simulink model "Simulink_linear_model"  (R2023b)
settings: Solver=ode45  StartTime=0.0  StopTime=10  MaxStep=0.01  RelTol=1e-3
values from neighbouring files (symbols this model uses):
  A = [0, 1,                    0, 0 ... (first row only)    [LQR_for_simscape_multibody_simulation.m]    (also in LQR_for_simulink.m)
  B = [0; (m*lc^2+J)/Delta; 0; -m*lc/Delta]    [LQR_for_simscape_multibody_simulation.m]    (also in LQR_for_simulink.m)
  K_lqr = lqr(A, B, Q, R)    [LQR_for_simscape_multibody_simulation.m]    (also in LQR_for_simulink.m)
settings Model: Creator=amira  LastModifiedBy=amira
settings DataIOCC: ReturnWorkspaceOutputs=off

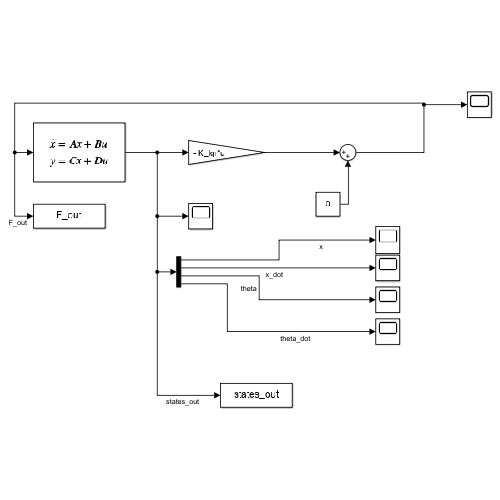
[thumbnail: Simulink's stored preview of the top-level diagram]
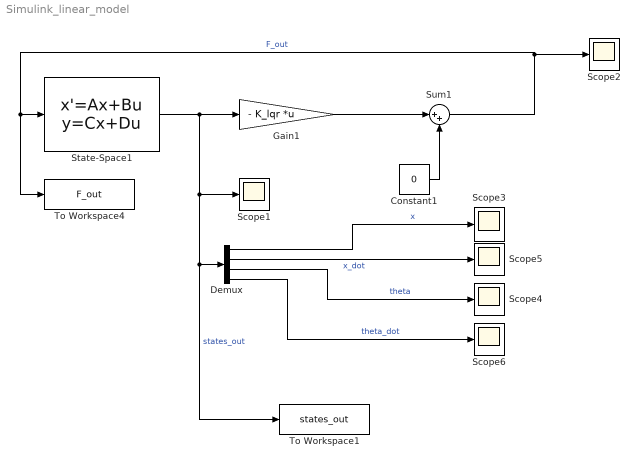
== system Simulink_linear_model ==
  Constant1 : Constant  Value=0
  Demux : Demux
  Gain1 : Gain  Gain=- K_lqr  Multiplication=Matrix(K*u)
  Scope{1..6} (6 alike) : Scope
  State-Space1 : StateSpace  A=A  B=B  C=eye(4)  D=zeros(4,1)  InitialCondition=[0; 0; 0.1; 0]  ParameterTunability=Unconstrained
  Sum1 : Sum  Inputs=|++
  To Workspace1 : ToWorkspace  VariableName=states_out  SampleTime=-1
  To Workspace4 : ToWorkspace  VariableName=F_out  SampleTime=-1
  wires:
  Constant1/1 -> Sum1/2
  Gain1/1 -> Sum1/1
  State-Space1/1 -> To Workspace1/1, Demux/1, Scope1/1, Gain1/1  "states_out"
  Demux/1 -> Scope3/1  "x"
  Demux/2 -> Scope5/1  "x_dot"
  Demux/3 -> Scope4/1  "theta"
  Demux/4 -> Scope6/1  "theta_dot"
  Sum1/1 -> Scope2/1, To Workspace4/1, State-Space1/1  "F_out"
